simulink model "ECU_Farol_Baixo_Model"  (R2024a)
settings: Solver=VariableStepAuto  StartTime=0.0  StopTime=10.0  RelTol=1e-3
settings Model: Creator=ec97883  LastModifiedBy=ec97883

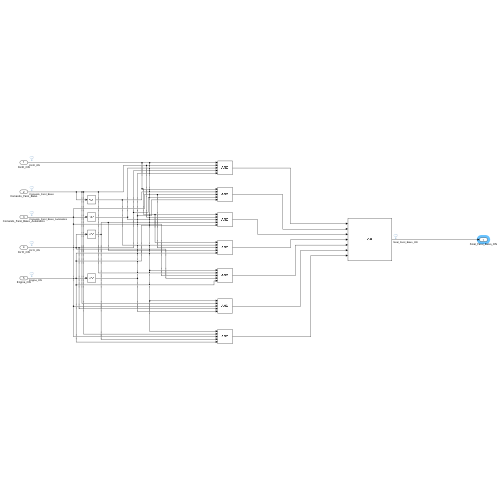
[thumbnail: Simulink's stored preview of the top-level diagram]
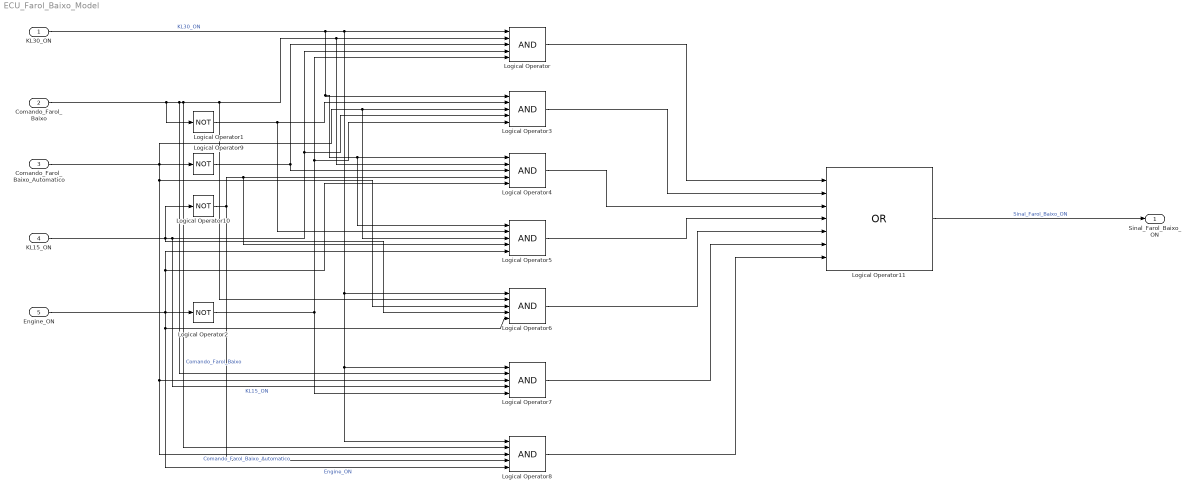
== system ECU_Farol_Baixo_Model ==
  KL30_ON : Inport  OutDataTypeStr=boolean  PortDimensions=1
  Comando_Farol_Baixo : Inport  Port=2  OutDataTypeStr=boolean  PortDimensions=1
  Comando_Farol_Baixo_Automatico : Inport  Port=3  OutDataTypeStr=boolean  PortDimensions=1
  KL15_ON : Inport  Port=4  OutDataTypeStr=boolean  PortDimensions=1
  Engine_ON : Inport  Port=5  OutDataTypeStr=boolean  PortDimensions=1
  Logical Operator{,3..8} (7 alike) : Logic  Inputs=5  AllPortsSameDT=off  OutDataTypeStr=boolean
  Logical Operator{1..2,9..10} (4 alike) : Logic  Operator=NOT  AllPortsSameDT=off  OutDataTypeStr=boolean
  Logical Operator11 : Logic  Operator=OR  Inputs=7  AllPortsSameDT=off  OutDataTypeStr=boolean
  Sinal_Farol_Baixo_ON : Outport  OutDataTypeStr=boolean  PortDimensions=1
  wires:
  Logical Operator/1 -> Logical Operator11/1
  Logical Operator3/1 -> Logical Operator11/2
  Logical Operator4/1 -> Logical Operator11/3
  Logical Operator5/1 -> Logical Operator11/4
  Logical Operator6/1 -> Logical Operator11/5
  Logical Operator7/1 -> Logical Operator11/6
  Logical Operator8/1 -> Logical Operator11/7
  KL30_ON/1 -> Logical Operator8/1, Logical Operator7/1, Logical Operator6/1, Logical Operator/1, Logical Operator5/1, Logical Operator4/1, Logical Operator3/1  "KL30_ON"
  Comando_Farol_Baixo/1 -> Logical Operator8/2, Logical Operator/2, Logical Operator4/2, Logical Operator6/2, Logical Operator7/2, Logical Operator1/1  "Comando_Farol_Baixo"
  Comando_Farol_Baixo_Automatico/1 -> Logical Operator8/3, Logical Operator7/3, Logical Operator6/3, Logical Operator5/3, Logical Operator3/3, Logical Operator9/1  "Comando_Farol_Baixo_Automatico"
  Logical Operator9/1 -> Logical Operator4/3, Logical Operator/3
  KL15_ON/1 -> Logical Operator/4, Logical Operator3/4, Logical Operator7/4, Logical Operator10/1, Logical Operator6/4  "KL15_ON"
  Engine_ON/1 -> Logical Operator6/5, Logical Operator8/5, Logical Operator4/5, Logical Operator5/5, Logical Operator2/1  "Engine_ON"
  Logical Operator2/1 -> Logical Operator7/5, Logical Operator3/5, Logical Operator/5
  Logical Operator1/1 -> Logical Operator5/2, Logical Operator3/2
  Logical Operator10/1 -> Logical Operator8/4, Logical Operator4/4, Logical Operator5/4
  Logical Operator11/1 -> Sinal_Farol_Baixo_ON/1  "Sinal_Farol_Baixo_ON"
